simulink model "test_datcom"  (R2016b)
settings: Solver=VariableStepAuto  StartTime=0.0  StopTime=10.0  RelTol=1e-3
undefined symbols (not defined in the file or in its folder): aero
libraries: aerolibasang x3, aerolib6dof2 x1, aerolibadyn x1, aerolibatmos2 x1
settings Model: Creator=notebook  LastModifiedBy=notebook

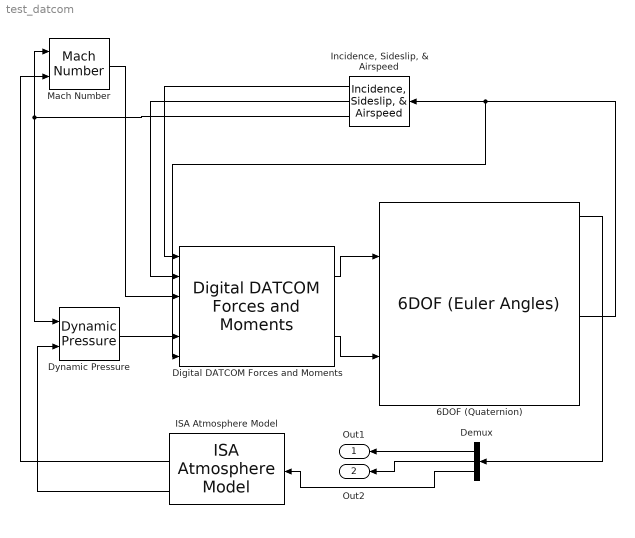
== system test_datcom ==
  6DOF (Quaternion) : aerolib6dof2/6DOF (Euler Angles)  units=Metric (MKS)  mtype=Fixed  rep=Quaternion  xme_0=[0 0 0]  Vm_0=[0 0 0]  eul_0=[0 0 0]  pm_0=[0 0 0]  mass_0=1.0  mass_e=0.5  mass_f=2.0  inertia=eye(3)  inertia_e=eye(3)  inertia_f=2*eye(3)  k_quat=1.0  vre_flag=on
  Demux : Demux  Outputs=3
  Digital DATCOM Forces and Moments : aerolibadyn/Digital DATCOM Forces and Moments  units=Metric (MKS)  dcase=aero{1}  fmode=Body  buildno=0  imethod=None - flat  emethod=None - clip  rmethod=Clip to Range  action=None
  Dynamic Pressure : aerolibasang/Dynamic Pressure
  ISA Atmosphere Model : aerolibatmos2/ISA Atmosphere Model  custom=off  g=9.80665  gamma=1.4  R=287.0531  L=0.0065  h_trop=11000  h_strat=20000  rho0=1.225  P0=101325  T0=288.15  h0=0
  "Incidence, Sideslip, & Airspeed" : aerolibasang/Incidence, Sideslip, & Airspeed
  Mach Number : aerolibasang/Mach Number
  Out1 : Outport
  Out2 : Outport  Port=2
  wires:
  Digital DATCOM Forces and Moments/2 -> 6DOF (Quaternion)/2
  Digital DATCOM Forces and Moments/1 -> 6DOF (Quaternion)/1
  6DOF (Quaternion)/5 -> Digital DATCOM Forces and Moments/6, "Incidence, Sideslip, & Airspeed"/1
  "Incidence, Sideslip, & Airspeed"/1 -> Digital DATCOM Forces and Moments/1
  "Incidence, Sideslip, & Airspeed"/2 -> Digital DATCOM Forces and Moments/2
  "Incidence, Sideslip, & Airspeed"/3 -> Mach Number/1, Dynamic Pressure/1
  Mach Number/1 -> Digital DATCOM Forces and Moments/3
  ISA Atmosphere Model/2 -> Mach Number/2
  Dynamic Pressure/1 -> Digital DATCOM Forces and Moments/5
  ISA Atmosphere Model/4 -> Dynamic Pressure/2
  6DOF (Quaternion)/1 -> Demux/1
  Demux/3 -> ISA Atmosphere Model/1
  Demux/1 -> Out1/1
  Demux/2 -> Out2/1
